simulink model "Display"  (R2014b)
settings: Solver=ode45  StartTime=0.0  StopTime=10.0  RelTol=1e-3
undefined symbols (not defined in the file): jet, maxNumSigns, template_detection_display, template_recognition_display
libraries: visiontextngfix x3, visionsinks x3, simulink x1
settings Model: Creator=Jackie  LastModifiedBy=Jackie

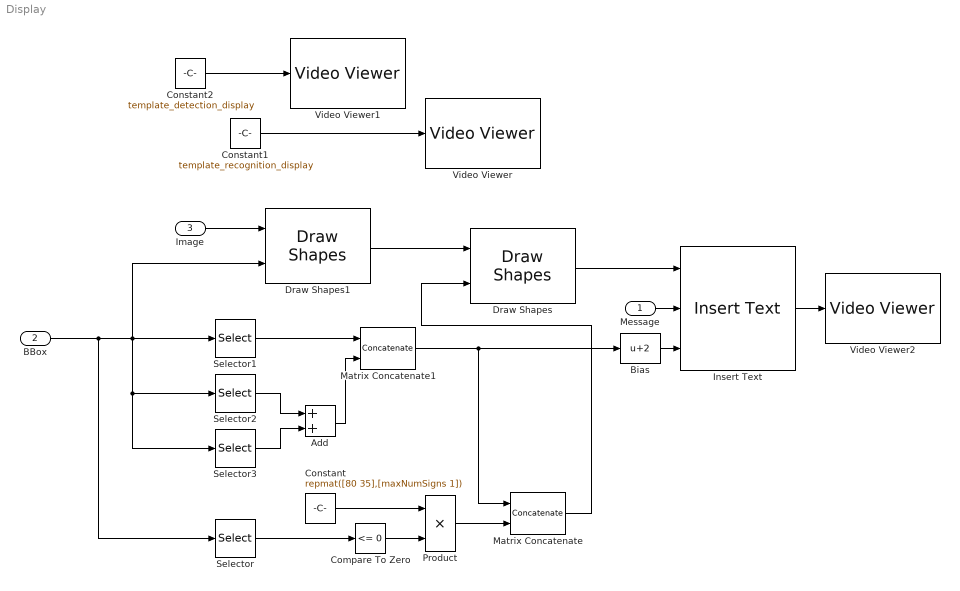
== system Display ==
  Message : Inport
  BBox : Inport  Port=2
  Image : Inport  Port=3
  Add : Sum
  Bias : Bias  Bias=2
  Compare To Zero : simulink/Logic and Bit Operations/Compare To Zero  relop=<=  OutDataTypeStr=boolean
  Constant : Constant  Value=repmat([80 35],[maxNumSigns 1])  VectorParams1D=off  OutDataTypeStr=single
  Constant1 : Constant  Value=template_recognition_display  OutDataTypeStr=single
  Constant2 : Constant  Value=template_detection_display  OutDataTypeStr=single
  Draw Shapes : visiontextngfix/Draw Shapes  shape=Rectangles  fill=on  lineWidth=1  fillClrSource=Specify via dialog  display=User-specified value  intensity=200  color=single([0 0 0])  opacity=single(1)  viewport=Entire image  antialiasing=off  inType=Obsolete  imagePorts=One multidimensional signal  prodOutputMode=Binary point scaling  prodOutputWordLength=32  prodOutputFracLength=14  memoryMode=Specify word length  memoryWordLength=16  memoryFracLength=14  roundingMode=Floor  overflowMode=off
  Draw Shapes1 : visiontextngfix/Draw Shapes  shape=Rectangles  fill=off  lineWidth=1  fillClrSource=Specify via dialog  display=User-specified value  intensity=200  color=[1 1 0]  opacity=0.6  viewport=Entire image  antialiasing=off  inType=Obsolete  imagePorts=One multidimensional signal  prodOutputMode=Binary point scaling  prodOutputWordLength=32  prodOutputFracLength=14  memoryMode=Specify word length  memoryWordLength=16  memoryFracLength=15  roundingMode=Floor  overflowMode=off
  Insert Text : visiontextngfix/Insert Text  inputType=Obsolete  theText='%s'  getTextLocFrom=Input port  textLoc=[1 1]  getTextColorFrom=Specify via dialog  textColor=[1 0 0]  getTextIntensityFrom=Specify via dialog  textIntensity=0  getTextOpacityFrom=Specify via dialog  textOpacity=1.0  dummyVar2=0  dummyVar3=0  dummyVar4=0  imagePorts=One multidimensional signal  isInputTransposed=off  fontFace=LucidaSansRegular  dummyVar1=0  blockFontSize=12  antiAliased=on
  Matrix Concatenate : Concatenate  Mode=Multidimensional array  ConcatenateDimension=2
  Matrix Concatenate1 : Concatenate  Mode=Multidimensional array  ConcatenateDimension=2
  Product : Product
  Selector : Selector  NumberOfDimensions=2  InputPortWidth=3  IndexOptions=Select all,Index vector (dialog)  Indices=[1 3],[3 4]  OutputSizes=1,1
  Selector1 : Selector  NumberOfDimensions=2  InputPortWidth=3  IndexOptions=Select all,Index vector (dialog)  Indices=[1 3],1  OutputSizes=1,1
  Selector2 : Selector  NumberOfDimensions=2  InputPortWidth=3  IndexOptions=Select all,Index vector (dialog)  Indices=[1 3],2  OutputSizes=1,1
  Selector3 : Selector  NumberOfDimensions=2  InputPortWidth=3  IndexOptions=Select all,Index vector (dialog)  Indices=[1 3],4  OutputSizes=1,1
  Video Viewer : visionsinks/Video Viewer  inputType=Obsolete7b  imagePorts=One multidimensional signal  useColorMap=off  colormapValue=jet(256)  specRange=off  minInputVal=0  maxInputVal=255  FigPos=[515 599 410 300]  AxisZoom=on  trueSizedOnce=off  OpenAtMdlStart=on  DefaultConfigurationName=vipscopes.VideoViewerScopeCfg
  Video Viewer1 : visionsinks/Video Viewer  inputType=Obsolete7b  imagePorts=One multidimensional signal  useColorMap=off  colormapValue=jet(256)  specRange=off  minInputVal=0  maxInputVal=255  FigPos=[515 599 410 300]  AxisZoom=on  trueSizedOnce=off  OpenAtMdlStart=on  DefaultConfigurationName=vipscopes.VideoViewerScopeCfg
  Video Viewer2 : visionsinks/Video Viewer  inputType=Obsolete7b  imagePorts=One multidimensional signal  useColorMap=off  colormapValue=jet(256)  specRange=off  minInputVal=0  maxInputVal=255  FigPos=[515 599 410 300]  AxisZoom=on  trueSizedOnce=off  OpenAtMdlStart=on  DefaultConfigurationName=vipscopes.VideoViewerScopeCfg
  wires:
  Insert Text/1 -> Video Viewer2/1
  Message/1 -> Insert Text/2
  Bias/1 -> Insert Text/3
  Draw Shapes/1 -> Insert Text/1
  Draw Shapes1/1 -> Draw Shapes/1
  Matrix Concatenate/1 -> Draw Shapes/2
  Matrix Concatenate1/1 -> Matrix Concatenate/1, Bias/1
  Product/1 -> Matrix Concatenate/2
  Compare To Zero/1 -> Product/2
  Selector2/1 -> Add/1
  Selector3/1 -> Add/2
  Selector1/1 -> Matrix Concatenate1/1
  Add/1 -> Matrix Concatenate1/2
  Selector/1 -> Compare To Zero/1
  Constant/1 -> Product/1
  Constant2/1 -> Video Viewer1/1
  Constant1/1 -> Video Viewer/1
  Image/1 -> Draw Shapes1/1
  BBox/1 -> Selector/1, Selector3/1, Selector2/1, Draw Shapes1/2, Selector1/1
